simulink model "sim_main_1"  (R2018b)
settings: Solver=ode23s  StartTime=0.0  StopTime=T_sweep  RelTol=1e-3
values from neighbouring files (symbols this model uses):
  dg = 0.65    [main_cntl.m]    (also in main_sys.m; main_sys_klm.m; main_tf_1.m; main_tf_10.m)
  dgs = 6    [main_cntl.m]    (also in main_sys.m; main_sys_klm.m; main_tf_1.m; main_tf_10.m)
  J_act = [0.000306 +  0.28200e-04]    [main_cntl.m]    (also in main_sys.m; main_sys_klm.m; main_tf_1.m; main_tf_10.m)
  Kg = 2.7e4    (= 27000)    [main_cntl.m]    (also in main_sys.m; main_sys_klm.m; main_tf_1.m; main_tf_10.m)
  rg = 160    [main_cntl.m]    (also in main_sys.m; main_sys_klm.m; main_tf_1.m; main_tf_10.m)
  Vel_mot_nom = 263    [main_cntl.m]    (also in main_sys.m; main_sys_klm.m; main_tf_1.m; main_tf_10.m)
undefined symbols (not defined in the file or in its folder): f_log, Jl, Jsint, ks
settings Model: Creator=eshojaei  LastModifiedBy=eshojaei
settings CodeAppCC: StateflowObjectComments=on

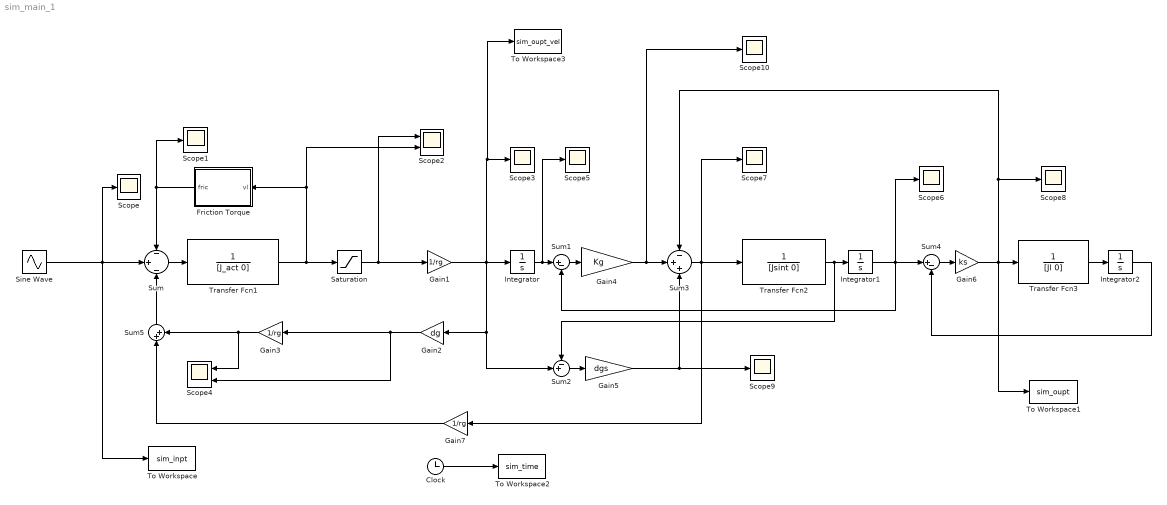
== system sim_main_1 ==
  Clock : Clock
  Friction Torque : MATLAB Function  TreatAsAtomicUnit=on
  Gain1 : Gain  Gain=1/rg
  Gain2 : Gain  Gain=dg
  Gain3 : Gain  Gain=1/rg
  Gain4 : Gain  Gain=Kg
  Gain5 : Gain  Gain=dgs
  Gain6 : Gain  Gain=ks
  Gain7 : Gain  Gain=1/rg
  Integrator : Integrator
  Integrator1 : Integrator
  Integrator2 : Integrator
  Saturation : Saturate  UpperLimit=Vel_mot_nom  LowerLimit=-Vel_mot_nom
  Scope{,1,3,5..10} (9 alike) : Scope
  Scope2 : Scope  NumInputPorts=2
  Scope4 : Scope  NumInputPorts=2
  Sine Wave : Sin  Amplitude=2  Frequency=5  SampleTime=0
  Sum : Sum  Inputs=-|+|-
  Sum1 : Sum  Inputs=|+-
  Sum2 : Sum  Inputs=-+|
  Sum3 : Sum  Inputs=-++
  Sum4 : Sum  Inputs=|+-
  Sum5 : Sum  Inputs=|++
  To Workspace : ToWorkspace  VariableName=sim_inpt  SaveFormat=Timeseries  SampleTime=1/f_log
  To Workspace1 : ToWorkspace  VariableName=sim_oupt  SaveFormat=Timeseries  SampleTime=1/f_log
  To Workspace2 : ToWorkspace  VariableName=sim_time  SaveFormat=Timeseries  SampleTime=1/f_log
  To Workspace3 : ToWorkspace  VariableName=sim_oupt_vel  SaveFormat=Timeseries  SampleTime=1/f_log
  Transfer Fcn1 : TransferFcn  Denominator=[J_act 0]
  Transfer Fcn2 : TransferFcn  Denominator=[Jsint 0]
  Transfer Fcn3 : TransferFcn  Denominator=[Jl 0]
  wires:
  Sine Wave/1 -> Scope/1, To Workspace/1, Sum/2
  Transfer Fcn1/1 -> Saturation/1, Friction Torque/1(vl), Scope2/2
  Saturation/1 -> Gain1/1, Scope2/1
  Friction Torque/1(fric) -> Sum/1, Scope1/1
  Sum/1 -> Transfer Fcn1/1
  Gain1/1 -> To Workspace3/1, Scope3/1, Integrator/1, Sum2/2, Gain2/1
  Gain2/1 -> Scope4/2, Gain3/1
  Gain3/1 -> Sum5/2, Scope4/1
  Integrator/1 -> Sum1/1, Scope5/1
  Sum1/1 -> Gain4/1
  Transfer Fcn2/1 -> Sum2/1, Integrator1/1
  Integrator1/1 -> Sum4/1, Scope6/1, Sum1/2
  Sum2/1 -> Gain5/1
  Sum3/1 -> Gain7/1, Transfer Fcn2/1, Scope7/1
  Sum4/1 -> Gain6/1
  Transfer Fcn3/1 -> Integrator2/1
  Integrator2/1 -> Sum4/2
  Sum5/1 -> Sum/3
  Clock/1 -> To Workspace2/1
  Gain7/1 -> Sum5/1
  Gain4/1 -> Scope10/1, Sum3/2
  Gain5/1 -> Sum3/3, Scope9/1
  Gain6/1 -> To Workspace1/1, Sum3/1, Scope8/1, Transfer Fcn3/1

== matlab function sim_main_1/Friction Torque ==
  data: vl input; fric output
function fric = fcn(vl)

    
   fric = (5981672325465929*vl)/147573952589676412928 + (7059617857129123*tanh((6072588977179245*vl)/36028797018963968))/144115188075855872 + (2558104915892175*tanh((5176012883402097*vl)/576460752303423488))/72057594037927936;
